simulink model "Seven_dof2024a_DK"  (R2025b)
settings: Solver=ode45  StartTime=0.0  StopTime=360  RelTol=1e-3
values from neighbouring files (symbols this model uses):
  Bf = 1.6    [Sensor_wz_u.m]    (also in unlinear_7DOF_Parameters.m)
  Br = 1.6    [Sensor_wz_u.m]    (also in unlinear_7DOF_Parameters.m)
  g = 9.8    [unlinear_7DOF_Parameters.m]
  hg = 0.5    [unlinear_7DOF_Parameters.m]
  i_sw = 20    [unlinear_7DOF_Parameters.m]
  L = Lf+Lr    (= 2.6)    [unlinear_7DOF_Parameters.m]
  Lf = 1.2    [Sensor_wz_u.m]    (also in unlinear_7DOF_Parameters.m)
  Lr = 1.4    [Sensor_wz_u.m]    (also in unlinear_7DOF_Parameters.m)
  mb = 1600    [unlinear_7DOF_Parameters.m]
  mw = (m-mb)/4    (= 41.25)    [unlinear_7DOF_Parameters.m]
  r = 0.354    [unlinear_7DOF_Parameters.m]
  u_fl = 0.3    [unlinear_7DOF_Parameters.m]
  u_fr = 0.8    [unlinear_7DOF_Parameters.m]
  u_rl = 0.3    [unlinear_7DOF_Parameters.m]
  u_rr = 0.8    [unlinear_7DOF_Parameters.m]
libraries: sharedTrackingLibrary x2, Solver_SF x1
settings Model: Creator=dzY  LastModifiedBy=odene
settings SolverCC: AlgebraicLoopSolver=TrustRegion
settings DataIOCC: LimitDataPoints=on  SaveFormat=Array  ReturnWorkspaceOutputs=off
settings OptimizationCC: BlockReduction=off  BooleanDataType=off  LifeSpan=inf
settings DebuggingCC: AlgebraicLoopMsg=none  SaveWithParameterizedLinksMsg=none  UnderspecifiedInitializationDetection=Classic  MergeDetectMultiDrivingBlocksExec=none  SignalResolutionControl=TryResolveAllWithWarning  UnconnectedInputMsg=warning  UnconnectedOutputMsg=warning  UnconnectedLineMsg=warning  SFUnexpectedBacktrackingDiag=warning  SFNoUnconditionalDefaultTransitionDiag=warning  SFExecutionAtInitializationDiag=none  ArithmeticOperatorsInVariantConditions=warning
settings HardwareCC: ProdBitPerPointer=32.0  ProdBitPerSizeT=32.0  ProdBitPerPtrDiffT=32.0  ProdLargestAtomicFloat=None  ProdIntDivRoundTo=Undefined  ProdEndianess=Unspecified  ProdWordSize=32.0  ProdHWDeviceType=32-bit Generic  TargetUnknown=on
settings ModelReferenceCC: EnableRefExpFcnMdlSchedulingChecks=on  PropagateSignalLabelsOutOfModel=off
settings SFSimCC: SimUseLocalCustomCode=off  CustomCodeUndefinedFunction=UseInterfaceOnly
settings RTWCC: RTWUseLocalCustomCode=off  GPUComputeCapability=3.5
settings CodeAppCC: StateflowObjectComments=on
settings GRTTargetCC: TargetLangStandard=C89/C90 (ANSI)
settings ConfigComp: CovMetricSettings=dw  CovSaveCumulativeToWorkspaceVar=on  CovSaveSingleToWorkspaceVar=on  CovExternalEMLEnable=off  CovSFcnEnable=off

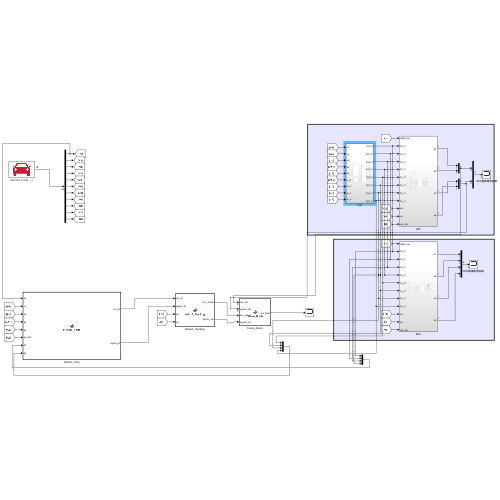
[thumbnail: Simulink's stored preview of the top-level diagram]
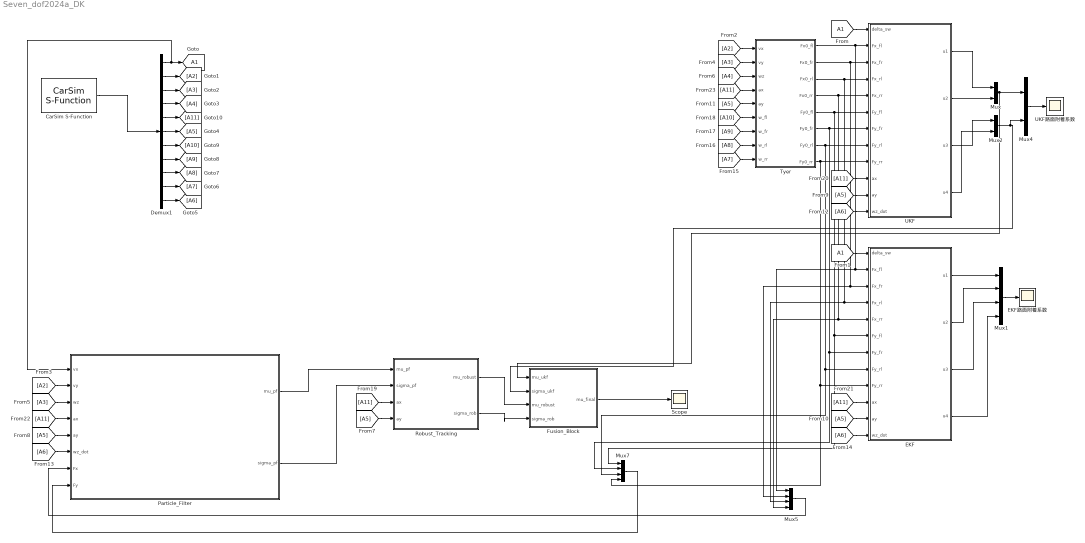
== system Seven_dof2024a_DK ==
  CarSim S-Function : Solver_SF/CarSim S-Function  Priority=1  VehicleCode=i_i  SIMFILE=simfile.sim
  Demux1 : Demux  Outputs=11
  EKF : Subsystem
  EKF路面附着系数 : Scope
      settings: ActiveDisplayYMinimum=0.13473  ActiveDisplayYMaximum=1.09614  DataLoggingSaveFormat=Array
  Fusion_Block : MATLAB Function  TreatAsAtomicUnit=on
  Mux : Mux  Inputs=2
  Mux1 : Mux
  Mux2 : Mux  Inputs=2
  Mux4 : Mux  Inputs=2
  Mux5 : Mux
  Mux7 : Mux
  Particle_Filter : MATLAB Function  TreatAsAtomicUnit=on
  Robust_Tracking : MATLAB Function  TreatAsAtomicUnit=on
  Scope : Scope
      settings: DataLoggingVariableName=ScopeData4
  Tyer : Subsystem
  UKF : Subsystem
  UKF路面附着系数 : Scope
      settings: ActiveDisplayYMinimum=0.13473  ActiveDisplayYMaximum=1.09614  DataLoggingSaveFormat=Array
  tag scope: A1=global
  wires:
  Mux4/1 -> UKF路面附着系数/1
  Tyer/1(Fx0_fl) -> Mux5/1, EKF/2(Fx_fl), UKF/2(Fx_fl)
  Tyer/2(Fx0_fr) -> Mux5/2, EKF/3(Fx_fr), UKF/3(Fx_fr)
  Tyer/3(Fx0_rl) -> Mux5/3, EKF/4(Fx_rl), UKF/4(Fx_rl)
  Tyer/4(Fx0_rr) -> Mux5/4, EKF/5(Fx_rr), UKF/5(Fx_rr)
  Tyer/5(Fy0_fl) -> Mux7/1, EKF/6(Fy_fl), UKF/6(Fy_fl)
  Tyer/6(Fy0_fr) -> Mux7/2, EKF/7(Fy_fr), UKF/7(Fy_fr)
  Tyer/7(Fy0_rl) -> Mux7/3, EKF/8(Fy_rl), UKF/8(Fy_rl)
  Tyer/8(Fy0_rr) -> Mux7/4, EKF/9(Fy_rr), UKF/9(Fy_rr)
  EKF/1(u1) -> Mux1/1
  EKF/2(u2) -> Mux1/2
  EKF/4(u4) -> Mux1/4
  EKF/3(u3) -> Mux1/3
  Mux1/1 -> EKF路面附着系数/1
  Fusion_Block/1(mu_final) -> Scope/1
  Mux5/1 -> Particle_Filter/7(Fx)
  Mux7/1 -> Particle_Filter/8(Fy)
  Particle_Filter/2(sigma_pf) -> Robust_Tracking/2(sigma_pf)
  Particle_Filter/1(mu_pf) -> Robust_Tracking/1(mu_pf)
  Robust_Tracking/2(sigma_rob) -> Fusion_Block/4(sigma_rob)
  Robust_Tracking/1(mu_robust) -> Fusion_Block/3(mu_robust)
  UKF/1(u1) -> Mux/1
  UKF/2(u2) -> Mux/2
  UKF/3(u3) -> Mux2/1
  UKF/4(u4) -> Mux2/2
  Mux/1 -> Fusion_Block/1(mu_ukf), Mux4/1
  Mux2/1 -> Fusion_Block/2(sigma_ukf), Mux4/2
  CarSim S-Function/1 -> Demux1/1
  Demux1/1 -> [A1], Particle_Filter/1(vx)
  [A1] -> UKF/1(delta_sw)
  [A1] -> EKF/1(delta_sw)
  Demux1/2 -> [A2]
  [A2] -> Tyer/1(vx)
  [A2] -> Particle_Filter/2(vy)
  Demux1/3 -> [A3]
  [A3] -> Tyer/2(vy)
  [A3] -> Particle_Filter/3(wz)
  Demux1/4 -> [A4]
  [A4] -> Tyer/3(wz)
  Demux1/6 -> [A5]
  [A5] -> Robust_Tracking/4(ay)
  [A5] -> Particle_Filter/5(ay)
  [A5] -> UKF/11(ay)
  [A5] -> EKF/11(ay)
  [A5] -> Tyer/5(ay)
  Demux1/11 -> [A6]
  [A6] -> UKF/12(wz_dot)
  [A6] -> Particle_Filter/6(wz_dot)
  [A6] -> EKF/12(wz_dot)
  Demux1/10 -> [A7]
  [A7] -> Tyer/9(w_rr)
  Demux1/9 -> [A8]
  [A8] -> Tyer/8(w_rl)
  Demux1/8 -> [A9]
  [A9] -> Tyer/7(w_fr)
  Demux1/7 -> [A10]
  [A10] -> Tyer/6(w_fl)
  Demux1/5 -> [A11]
  [A11] -> Robust_Tracking/3(ax)
  [A11] -> UKF/10(ax)
  [A11] -> EKF/10(ax)
  [A11] -> Particle_Filter/4(ax)
  [A11] -> Tyer/4(ax)

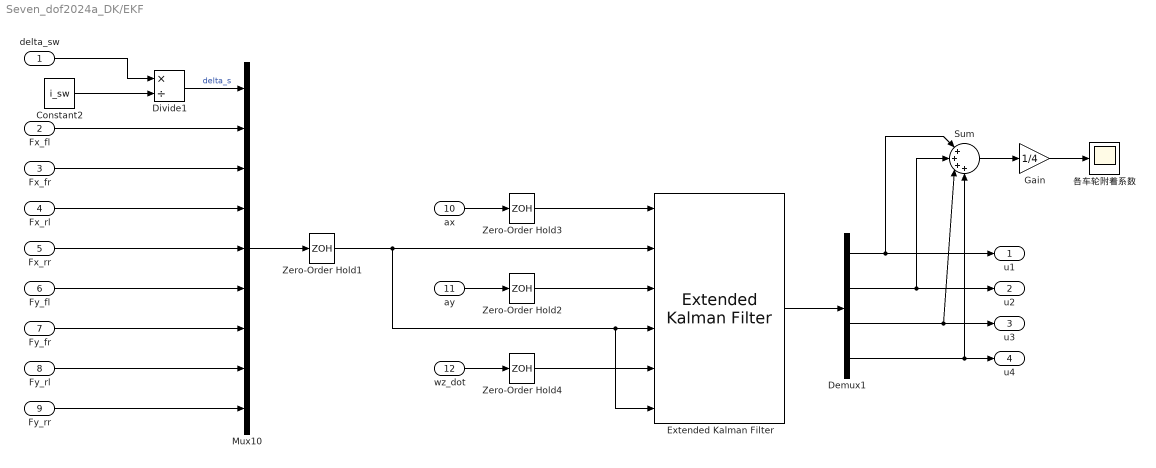
== system Seven_dof2024a_DK/EKF ==
  delta_sw : Inport
  Fx_fl : Inport  Port=2
  Fx_fr : Inport  Port=3
  Fx_rl : Inport  Port=4
  Fx_rr : Inport  Port=5
  Fy_fl : Inport  Port=6
  Fy_fr : Inport  Port=7
  Fy_rl : Inport  Port=8
  Fy_rr : Inport  Port=9
  ax : Inport  Port=10
  ay : Inport  Port=11
  wz_dot : Inport  Port=12
  Constant2 : Constant  Value=i_sw
  Demux1 : Demux
  Divide1 : Product  Inputs=*/
  Extended Kalman Filter : sharedTrackingLibrary/Extended Kalman Filter  StateTransitionFcn=LinearState_u  HasStateTransitionJacobianFcn=off  HasAdditiveProcessNoise=Additive  ProcessNoise=diag([0.1 0.1 0.1 0.1])  HasTimeVaryingProcessNoise=off  HasStateTransitionFcnExtraArgument=0  InitialState=[1;1; 1; 1]  InitialStateCovariance=1e-4  MeasurementFcn1=Sensor_ax_u  HasMeasurementJacobianFcn1=off  HasMeasurementEnablePort1=off  HasAdditiveMeasurementNoise1=Additive  MeasurementNoise1=0.0001  HasTimeVaryingMeasurementNoise1=off  HasMeasurementFcnExtraArgument1=1  HasMeasurementWrapping1=off  MeasurementFcn2=Sensor_ay_u  HasMeasurementJacobianFcn2=off  HasMeasurementEnablePort2=off  HasAdditiveMeasurementNoise2=Additive  MeasurementNoise2=0.0001  HasTimeVaryingMeasurementNoise2=off  HasMeasurementFcnExtraArgument2=1  HasMeasurementWrapping2=off  MeasurementFcn3=Sensor_wz_u  HasMeasurementJacobianFcn3=off  HasMeasurementEnablePort3=off  HasAdditiveMeasurementNoise3=Additive  MeasurementNoise3=0.0001  HasTimeVaryingMeasurementNoise3=off  HasMeasurementFcnExtraArgument3=1  HasMeasurementWrapping3=off  MeasurementFcn4=myMeasurementFcn  HasMeasurementJacobianFcn4=off  HasMeasurementEnablePort4=off  HasAdditiveMeasurementNoise4=Additive  MeasurementNoise4=1  HasTimeVaryingMeasurementNoise4=off  HasMeasurementFcnExtraArgument4=0  HasMeasurementWrapping4=off  MeasurementFcn5=myMeasurementFcn  HasMeasurementJacobianFcn5=off  HasMeasurementEnablePort5=off  HasAdditiveMeasurementNoise5=Additive  MeasurementNoise5=1  HasTimeVaryingMeasurementNoise5=off  HasMeasurementFcnExtraArgument5=0  HasMeasurementWrapping5=off  EnableMultirate=on  StateTransitionFcnSampleTime=0.01  MeasurementFcn1SampleTime=0.01  MeasurementFcn2SampleTime=0.01  MeasurementFcn3SampleTime=0.01  MeasurementFcn4SampleTime=1  MeasurementFcn5SampleTime=1  UseCurrentEstimator=on  OutputStateCovariance=off  DataType=double  SampleTime=0.01  NumberOfMeasurements=3
  Gain : Gain  Gain=1/4
  Mux10 : Mux  Inputs=9
  Sum : Sum  Inputs=|++++
  Zero-Order Hold{1..4} (4 alike) : ZeroOrderHold  SampleTime=0.01
  各车轮附着系数 : Scope
      settings: ActiveDisplayYMinimum=0.54572  ActiveDisplayYMaximum=0.55343
  u1 : Outport  VectorParamsAs1DForOutWhenUnconnected=off
  u2 : Outport  Port=2  VectorParamsAs1DForOutWhenUnconnected=off
  u3 : Outport  Port=3  VectorParamsAs1DForOutWhenUnconnected=off
  u4 : Outport  Port=4  VectorParamsAs1DForOutWhenUnconnected=off
  wires:
  Gain/1 -> 各车轮附着系数/1
  Sum/1 -> Gain/1
  Zero-Order Hold3/1 -> Extended Kalman Filter/1
  Zero-Order Hold2/1 -> Extended Kalman Filter/3
  Demux1/4 -> Sum/4, u4/1
  Zero-Order Hold1/1 -> Extended Kalman Filter/2, Extended Kalman Filter/6, Extended Kalman Filter/4
  Fy_rr/1 -> Mux10/9
  Fy_rl/1 -> Mux10/8
  Fy_fr/1 -> Mux10/7
  Fy_fl/1 -> Mux10/6
  Fx_rr/1 -> Mux10/5
  Fx_rl/1 -> Mux10/4
  Fx_fr/1 -> Mux10/3
  Fx_fl/1 -> Mux10/2
  Zero-Order Hold4/1 -> Extended Kalman Filter/5
  wz_dot/1 -> Zero-Order Hold4/1
  ay/1 -> Zero-Order Hold2/1
  ax/1 -> Zero-Order Hold3/1
  Constant2/1 -> Divide1/2
  delta_sw/1 -> Divide1/1
  Extended Kalman Filter/1 -> Demux1/1
  Mux10/1 -> Zero-Order Hold1/1
  Divide1/1 -> Mux10/1  "delta_s"
  Demux1/1 -> u1/1, Sum/1
  Demux1/3 -> Sum/3, u3/1
  Demux1/2 -> u2/1, Sum/2

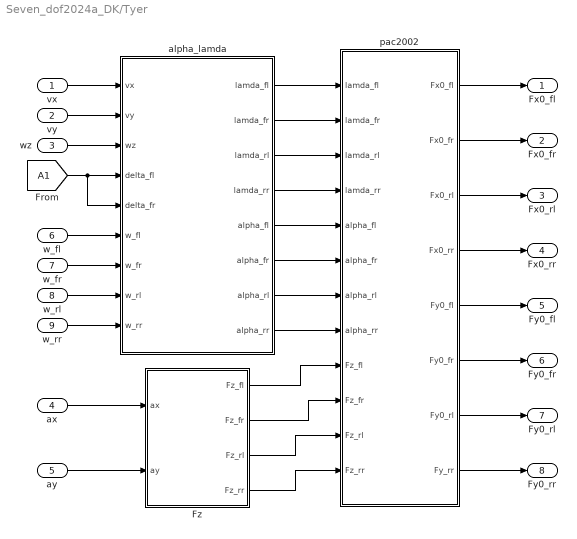
== system Seven_dof2024a_DK/Tyer ==
  vx : Inport
  vy : Inport  Port=2
  wz : Inport  Port=3
  ax : Inport  Port=4
  ay : Inport  Port=5
  w_fl : Inport  Port=6
  w_fr : Inport  Port=7
  w_rl : Inport  Port=8
  w_rr : Inport  Port=9
  Fz : Subsystem
  alpha_lamda : Subsystem
  pac2002 : Subsystem
  Fx0_fl : Outport  VectorParamsAs1DForOutWhenUnconnected=off
  Fx0_fr : Outport  Port=2  VectorParamsAs1DForOutWhenUnconnected=off
  Fx0_rl : Outport  Port=3  VectorParamsAs1DForOutWhenUnconnected=off
  Fx0_rr : Outport  Port=4  VectorParamsAs1DForOutWhenUnconnected=off
  Fy0_fl : Outport  Port=5  VectorParamsAs1DForOutWhenUnconnected=off
  Fy0_fr : Outport  Port=6  VectorParamsAs1DForOutWhenUnconnected=off
  Fy0_rl : Outport  Port=7  VectorParamsAs1DForOutWhenUnconnected=off
  Fy0_rr : Outport  Port=8  VectorParamsAs1DForOutWhenUnconnected=off
  wires:
  ay/1 -> Fz/2(ay)
  ax/1 -> Fz/1(ax)
  [A1] -> alpha_lamda/5(delta_fr), alpha_lamda/4(delta_fl)
  vx/1 -> alpha_lamda/1(vx)
  vy/1 -> alpha_lamda/2(vy)
  wz/1 -> alpha_lamda/3(wz)
  w_fl/1 -> alpha_lamda/6(w_fl)
  w_fr/1 -> alpha_lamda/7(w_fr)
  w_rl/1 -> alpha_lamda/8(w_rl)
  w_rr/1 -> alpha_lamda/9(w_rr)
  alpha_lamda/1(lamda_fl) -> pac2002/1(lamda_fl)
  alpha_lamda/2(lamda_fr) -> pac2002/2(lamda_fr)
  alpha_lamda/3(lamda_rl) -> pac2002/3(lamda_rl)
  alpha_lamda/4(lamda_rr) -> pac2002/4(lamda_rr)
  alpha_lamda/5(alpha_fl) -> pac2002/5(alpha_fl)
  alpha_lamda/6(alpha_fr) -> pac2002/6(alpha_fr)
  alpha_lamda/7(alpha_rl) -> pac2002/7(alpha_rl)
  alpha_lamda/8(alpha_rr) -> pac2002/8(alpha_rr)
  Fz/1(Fz_fl) -> pac2002/9(Fz_fl)
  Fz/2(Fz_fr) -> pac2002/10(Fz_fr)
  Fz/3(Fz_rl) -> pac2002/11(Fz_rl)
  Fz/4(Fz_rr) -> pac2002/12(Fz_rr)
  pac2002/1(Fx0_fl) -> Fx0_fl/1
  pac2002/2(Fx0_fr) -> Fx0_fr/1
  pac2002/3(Fx0_rl) -> Fx0_rl/1
  pac2002/4(Fx0_rr) -> Fx0_rr/1
  pac2002/5(Fy0_fl) -> Fy0_fl/1
  pac2002/6(Fy0_fr) -> Fy0_fr/1
  pac2002/7(Fy0_rl) -> Fy0_rl/1
  pac2002/8(Fy_rr) -> Fy0_rr/1

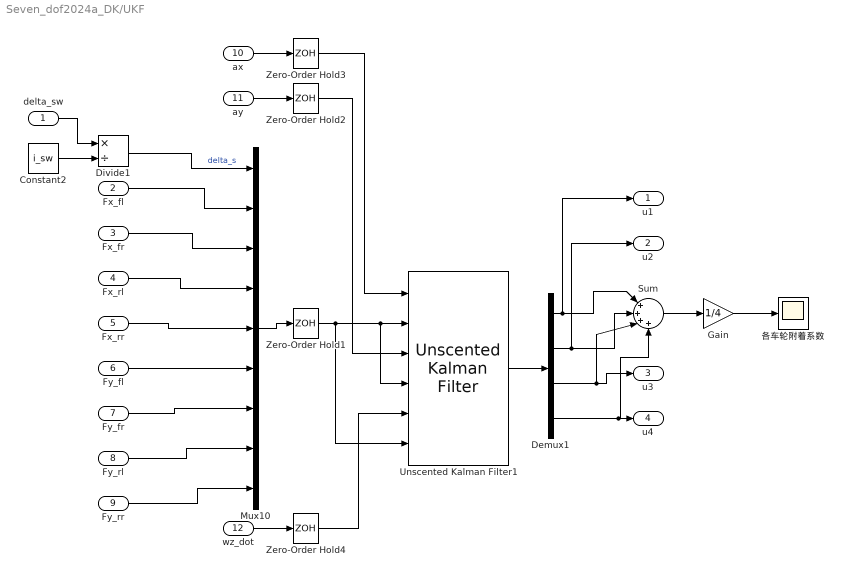
== system Seven_dof2024a_DK/UKF ==
  delta_sw : Inport
  Fx_fl : Inport  Port=2
  Fx_fr : Inport  Port=3
  Fx_rl : Inport  Port=4
  Fx_rr : Inport  Port=5
  Fy_fl : Inport  Port=6
  Fy_fr : Inport  Port=7
  Fy_rl : Inport  Port=8
  Fy_rr : Inport  Port=9
  ax : Inport  Port=10
  ay : Inport  Port=11
  wz_dot : Inport  Port=12
  Constant2 : Constant  Value=i_sw
  Demux1 : Demux
  Divide1 : Product  Inputs=*/
  Gain : Gain  Gain=1/4
  Mux10 : Mux  Inputs=9
  Sum : Sum  Inputs=|++++
  Unscented Kalman Filter1 : sharedTrackingLibrary/Unscented Kalman Filter  StateTransitionFcn=LinearState_u  HasAdditiveProcessNoise=Additive  ProcessNoise=diag([0.1 0.1 0.1 0.1])  HasTimeVaryingProcessNoise=off  HasStateTransitionFcnExtraArgument=0  InitialState=[1;1; 1; 1]  InitialStateCovariance=1e-4  Alpha=1e-3  Beta=2  Kappa=0  MeasurementFcn1=Sensor_ax_u  HasMeasurementEnablePort1=off  HasAdditiveMeasurementNoise1=Additive  MeasurementNoise1=0.0001  HasTimeVaryingMeasurementNoise1=off  HasMeasurementFcnExtraArgument1=1  HasMeasurementWrapping1=off  MeasurementFcn2=Sensor_ay_u  HasMeasurementEnablePort2=off  HasAdditiveMeasurementNoise2=Additive  MeasurementNoise2=0.0001  HasTimeVaryingMeasurementNoise2=off  HasMeasurementFcnExtraArgument2=1  HasMeasurementWrapping2=off  MeasurementFcn3=Sensor_wz_u  HasMeasurementEnablePort3=off  HasAdditiveMeasurementNoise3=Additive  MeasurementNoise3=0.0001  HasTimeVaryingMeasurementNoise3=off  HasMeasurementFcnExtraArgument3=1  HasMeasurementWrapping3=off  MeasurementFcn4=myMeasurementFcn  HasMeasurementEnablePort4=off  HasAdditiveMeasurementNoise4=Additive  MeasurementNoise4=1  HasTimeVaryingMeasurementNoise4=off  HasMeasurementFcnExtraArgument4=0  HasMeasurementWrapping4=off  MeasurementFcn5=myMeasurementFcn  HasMeasurementEnablePort5=off  HasAdditiveMeasurementNoise5=Additive  MeasurementNoise5=1  HasTimeVaryingMeasurementNoise5=off  HasMeasurementFcnExtraArgument5=0  HasMeasurementWrapping5=off  EnableMultirate=on  StateTransitionFcnSampleTime=0.01  MeasurementFcn1SampleTime=0.01  MeasurementFcn2SampleTime=0.01  MeasurementFcn3SampleTime=0.01  MeasurementFcn4SampleTime=1  MeasurementFcn5SampleTime=1  UseCurrentEstimator=on  OutputStateCovariance=off  DataType=double  SampleTime=1  NumberOfMeasurements=3
      link override Correct3/MATLAB System: SimulateUsing=Interpreted execution
  Zero-Order Hold{1..4} (4 alike) : ZeroOrderHold  SampleTime=0.01
  各车轮附着系数 : Scope
      settings: ActiveDisplayYMinimum=0.49277  ActiveDisplayYMaximum=1.05636
  u1 : Outport  VectorParamsAs1DForOutWhenUnconnected=off
  u2 : Outport  Port=2  VectorParamsAs1DForOutWhenUnconnected=off
  u3 : Outport  Port=3  VectorParamsAs1DForOutWhenUnconnected=off
  u4 : Outport  Port=4  VectorParamsAs1DForOutWhenUnconnected=off
  wires:
  Fx_fr/1 -> Mux10/3
  delta_sw/1 -> Divide1/1
  Fx_rr/1 -> Mux10/5
  Constant2/1 -> Divide1/2
  Zero-Order Hold4/1 -> Unscented Kalman Filter1/5
  Fy_fl/1 -> Mux10/6
  Fx_rl/1 -> Mux10/4
  Divide1/1 -> Mux10/1  "delta_s"
  Fx_fl/1 -> Mux10/2
  Fy_fr/1 -> Mux10/7
  Fy_rl/1 -> Mux10/8
  Fy_rr/1 -> Mux10/9
  ax/1 -> Zero-Order Hold3/1
  Sum/1 -> Gain/1
  ay/1 -> Zero-Order Hold2/1
  wz_dot/1 -> Zero-Order Hold4/1
  Zero-Order Hold3/1 -> Unscented Kalman Filter1/1
  Zero-Order Hold2/1 -> Unscented Kalman Filter1/3
  Zero-Order Hold1/1 -> Unscented Kalman Filter1/4, Unscented Kalman Filter1/2, Unscented Kalman Filter1/6
  Demux1/4 -> Sum/4, u4/1
  Unscented Kalman Filter1/1 -> Demux1/1
  Demux1/1 -> Sum/1, u1/1
  Demux1/2 -> Sum/2, u2/1
  Demux1/3 -> Sum/3, u3/1
  Gain/1 -> 各车轮附着系数/1
  Mux10/1 -> Zero-Order Hold1/1

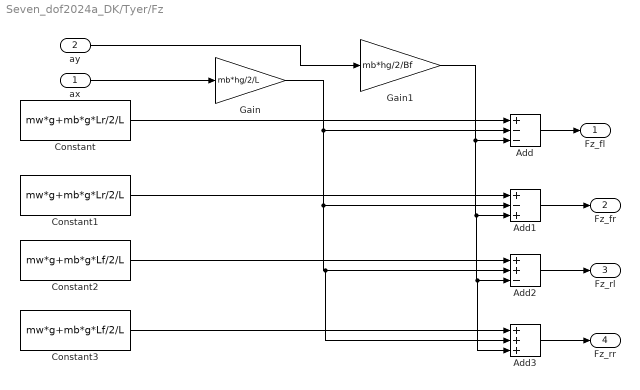
== system Seven_dof2024a_DK/Tyer/Fz ==
  ax : Inport
  ay : Inport  Port=2
  Add : Sum  Inputs=+--
  Add1 : Sum  Inputs=+-+
  Add2 : Sum  Inputs=++-
  Add3 : Sum  Inputs=+++
  Constant : Constant  Value=mw*g+mb*g*Lr/2/L
  Constant1 : Constant  Value=mw*g+mb*g*Lr/2/L
  Constant2 : Constant  Value=mw*g+mb*g*Lf/2/L
  Constant3 : Constant  Value=mw*g+mb*g*Lf/2/L
  Gain : Gain  Gain=mb*hg/2/L
  Gain1 : Gain  Gain=mb*hg/2/Bf
  Fz_fl : Outport  VectorParamsAs1DForOutWhenUnconnected=off
  Fz_fr : Outport  Port=2  VectorParamsAs1DForOutWhenUnconnected=off
  Fz_rl : Outport  Port=3  VectorParamsAs1DForOutWhenUnconnected=off
  Fz_rr : Outport  Port=4  VectorParamsAs1DForOutWhenUnconnected=off
  wires:
  Constant1/1 -> Add1/1
  Constant2/1 -> Add2/1
  Constant/1 -> Add/1
  Gain/1 -> Add3/2, Add2/2, Add1/2, Add/2
  Gain1/1 -> Add3/3, Add2/3, Add1/3, Add/3
  Constant3/1 -> Add3/1
  ay/1 -> Gain1/1
  ax/1 -> Gain/1
  Add3/1 -> Fz_rr/1
  Add2/1 -> Fz_rl/1
  Add1/1 -> Fz_fr/1
  Add/1 -> Fz_fl/1

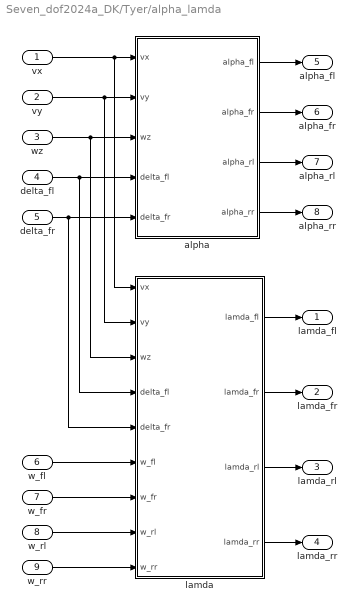
== system Seven_dof2024a_DK/Tyer/alpha_lamda ==
  vx : Inport
  vy : Inport  Port=2
  wz : Inport  Port=3
  delta_fl : Inport  Port=4
  delta_fr : Inport  Port=5
  w_fl : Inport  Port=6
  w_fr : Inport  Port=7
  w_rl : Inport  Port=8
  w_rr : Inport  Port=9
  alpha : Subsystem
  lamda : Subsystem
  lamda_fl : Outport  VectorParamsAs1DForOutWhenUnconnected=off
  lamda_fr : Outport  Port=2  VectorParamsAs1DForOutWhenUnconnected=off
  lamda_rl : Outport  Port=3  VectorParamsAs1DForOutWhenUnconnected=off
  lamda_rr : Outport  Port=4  VectorParamsAs1DForOutWhenUnconnected=off
  alpha_fl : Outport  Port=5  VectorParamsAs1DForOutWhenUnconnected=off
  alpha_fr : Outport  Port=6  VectorParamsAs1DForOutWhenUnconnected=off
  alpha_rl : Outport  Port=7  VectorParamsAs1DForOutWhenUnconnected=off
  alpha_rr : Outport  Port=8  VectorParamsAs1DForOutWhenUnconnected=off
  wires:
  lamda/3(lamda_rl) -> lamda_rl/1
  lamda/4(lamda_rr) -> lamda_rr/1
  lamda/2(lamda_fr) -> lamda_fr/1
  lamda/1(lamda_fl) -> lamda_fl/1
  w_rr/1 -> lamda/9(w_rr)
  w_rl/1 -> lamda/8(w_rl)
  w_fr/1 -> lamda/7(w_fr)
  w_fl/1 -> lamda/6(w_fl)
  delta_fr/1 -> alpha/5(delta_fr), lamda/5(delta_fr)
  delta_fl/1 -> alpha/4(delta_fl), lamda/4(delta_fl)
  wz/1 -> alpha/3(wz), lamda/3(wz)
  vy/1 -> alpha/2(vy), lamda/2(vy)
  vx/1 -> alpha/1(vx), lamda/1(vx)
  alpha/4(alpha_rr) -> alpha_rr/1
  alpha/3(alpha_rl) -> alpha_rl/1
  alpha/2(alpha_fr) -> alpha_fr/1
  alpha/1(alpha_fl) -> alpha_fl/1

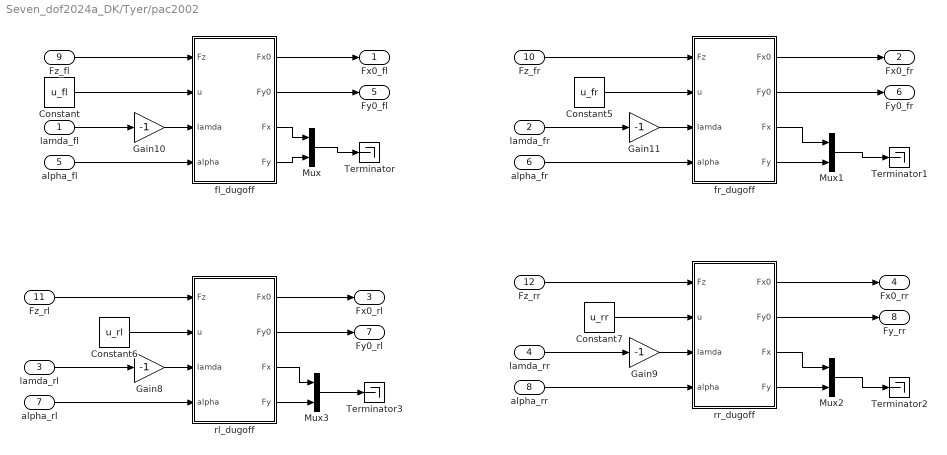
== system Seven_dof2024a_DK/Tyer/pac2002 ==
  lamda_fl : Inport
  lamda_fr : Inport  Port=2
  lamda_rl : Inport  Port=3
  lamda_rr : Inport  Port=4
  alpha_fl : Inport  Port=5
  alpha_fr : Inport  Port=6
  alpha_rl : Inport  Port=7
  alpha_rr : Inport  Port=8
  Fz_fl : Inport  Port=9
  Fz_fr : Inport  Port=10
  Fz_rl : Inport  Port=11
  Fz_rr : Inport  Port=12
  Constant : Constant  Value=u_fl
  Constant5 : Constant  Value=u_fr
  Constant6 : Constant  Value=u_rl
  Constant7 : Constant  Value=u_rr
  Gain{8..11} (4 alike) : Gain  Gain=-1
  Mux{,1..3} (4 alike) : Mux  Inputs=2
  Terminator{,1..3} (4 alike) : Terminator
  fl_dugoff : MATLAB Function  TreatAsAtomicUnit=on
  fr_dugoff : MATLAB Function  TreatAsAtomicUnit=on
  rl_dugoff : MATLAB Function  TreatAsAtomicUnit=on
  rr_dugoff : MATLAB Function  TreatAsAtomicUnit=on
  Fx0_fl : Outport  VectorParamsAs1DForOutWhenUnconnected=off
  Fx0_fr : Outport  Port=2  VectorParamsAs1DForOutWhenUnconnected=off
  Fx0_rl : Outport  Port=3  VectorParamsAs1DForOutWhenUnconnected=off
  Fx0_rr : Outport  Port=4  VectorParamsAs1DForOutWhenUnconnected=off
  Fy0_fl : Outport  Port=5  VectorParamsAs1DForOutWhenUnconnected=off
  Fy0_fr : Outport  Port=6  VectorParamsAs1DForOutWhenUnconnected=off
  Fy0_rl : Outport  Port=7  VectorParamsAs1DForOutWhenUnconnected=off
  Fy_rr : Outport  Port=8  VectorParamsAs1DForOutWhenUnconnected=off
  wires:
  alpha_fl/1 -> fl_dugoff/4(alpha)
  Fz_fl/1 -> fl_dugoff/1(Fz)
  Fz_rl/1 -> rl_dugoff/1(Fz)
  alpha_rr/1 -> rr_dugoff/4(alpha)
  Fz_rr/1 -> rr_dugoff/1(Fz)
  Constant/1 -> fl_dugoff/2(u)
  Fz_fr/1 -> fr_dugoff/1(Fz)
  Constant5/1 -> fr_dugoff/2(u)
  alpha_fr/1 -> fr_dugoff/4(alpha)
  Constant6/1 -> rl_dugoff/2(u)
  Constant7/1 -> rr_dugoff/2(u)
  lamda_fr/1 -> Gain11/1
  lamda_rl/1 -> Gain8/1
  lamda_rr/1 -> Gain9/1
  lamda_fl/1 -> Gain10/1
  fl_dugoff/1(Fx0) -> Fx0_fl/1
  rl_dugoff/1(Fx0) -> Fx0_rl/1
  fl_dugoff/2(Fy0) -> Fy0_fl/1
  fr_dugoff/2(Fy0) -> Fy0_fr/1
  rl_dugoff/2(Fy0) -> Fy0_rl/1
  rr_dugoff/2(Fy0) -> Fy_rr/1
  rr_dugoff/1(Fx0) -> Fx0_rr/1
  alpha_rl/1 -> rl_dugoff/4(alpha)
  Gain8/1 -> rl_dugoff/3(lamda)
  Gain9/1 -> rr_dugoff/3(lamda)
  Gain10/1 -> fl_dugoff/3(lamda)
  Gain11/1 -> fr_dugoff/3(lamda)
  fr_dugoff/1(Fx0) -> Fx0_fr/1
  fl_dugoff/3(Fx) -> Mux/1
  fl_dugoff/4(Fy) -> Mux/2
  Mux/1 -> Terminator/1
  Mux1/1 -> Terminator1/1
  fr_dugoff/3(Fx) -> Mux1/1
  fr_dugoff/4(Fy) -> Mux1/2
  rr_dugoff/3(Fx) -> Mux2/1
  rr_dugoff/4(Fy) -> Mux2/2
  Mux2/1 -> Terminator2/1
  rl_dugoff/3(Fx) -> Mux3/1
  rl_dugoff/4(Fy) -> Mux3/2
  Mux3/1 -> Terminator3/1

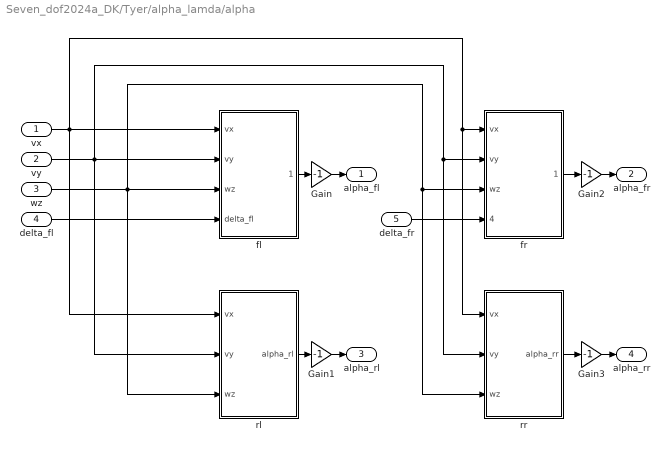
== system Seven_dof2024a_DK/Tyer/alpha_lamda/alpha ==
  vx : Inport
  vy : Inport  Port=2
  wz : Inport  Port=3
  delta_fl : Inport  Port=4
  delta_fr : Inport  Port=5
  Gain{,1..3} (4 alike) : Gain  Gain=-1
  fl : Subsystem
  fr : Subsystem
  rl : Subsystem
  rr : Subsystem
  alpha_fl : Outport  VectorParamsAs1DForOutWhenUnconnected=off
  alpha_fr : Outport  Port=2  VectorParamsAs1DForOutWhenUnconnected=off
  alpha_rl : Outport  Port=3  VectorParamsAs1DForOutWhenUnconnected=off
  alpha_rr : Outport  Port=4  VectorParamsAs1DForOutWhenUnconnected=off
  wires:
  delta_fr/1 -> fr/4(delta_fr)
  delta_fl/1 -> fl/4(delta_fl)
  vy/1 -> rl/2(vy), fl/2(vy), fr/2(vy), rr/2(vy)
  vx/1 -> rl/1(vx), fl/1(vx), fr/1(vx), rr/1(vx)
  wz/1 -> rl/3(wz), fr/3(wz), rr/3(wz), fl/3(wz)
  fl/1(alpha_fl) -> Gain/1
  Gain/1 -> alpha_fl/1
  rl/1(alpha_rl) -> Gain1/1
  Gain1/1 -> alpha_rl/1
  fr/1(alpha_fr) -> Gain2/1
  Gain2/1 -> alpha_fr/1
  rr/1(alpha_rr) -> Gain3/1
  Gain3/1 -> alpha_rr/1

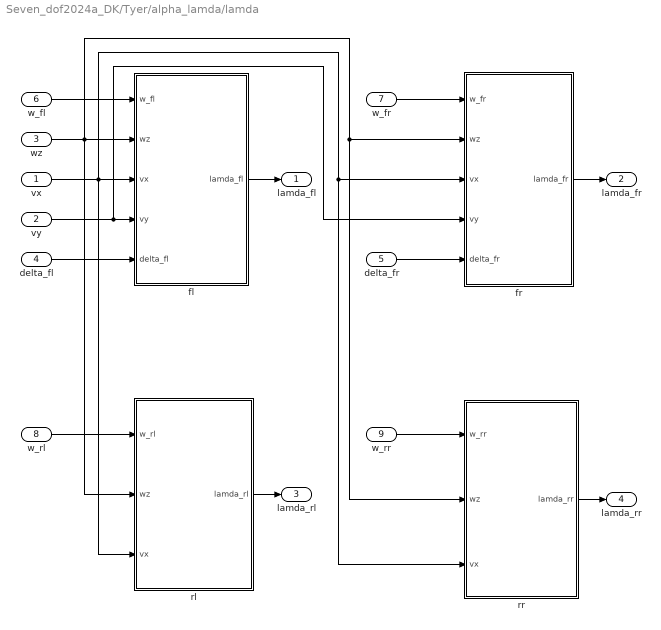
== system Seven_dof2024a_DK/Tyer/alpha_lamda/lamda ==
  vx : Inport
  vy : Inport  Port=2
  wz : Inport  Port=3
  delta_fl : Inport  Port=4
  delta_fr : Inport  Port=5
  w_fl : Inport  Port=6
  w_fr : Inport  Port=7
  w_rl : Inport  Port=8
  w_rr : Inport  Port=9
  fl : Subsystem
  fr : Subsystem
  rl : Subsystem
  rr : Subsystem
  lamda_fl : Outport  VectorParamsAs1DForOutWhenUnconnected=off
  lamda_fr : Outport  Port=2  VectorParamsAs1DForOutWhenUnconnected=off
  lamda_rl : Outport  Port=3  VectorParamsAs1DForOutWhenUnconnected=off
  lamda_rr : Outport  Port=4  VectorParamsAs1DForOutWhenUnconnected=off
  wires:
  fr/1(lamda_fr) -> lamda_fr/1
  rr/1(lamda_rr) -> lamda_rr/1
  w_rl/1 -> rl/1(w_rl)
  w_rr/1 -> rr/1(w_rr)
  w_fr/1 -> fr/1(w_fr)
  delta_fr/1 -> fr/5(delta_fr)
  delta_fl/1 -> fl/5(delta_fl)
  vy/1 -> fl/4(vy), fr/4(vy)
  vx/1 -> fl/3(vx), fr/3(vx), rr/3(vx), rl/3(vx)
  wz/1 -> fl/2(wz), fr/2(wz), rr/2(wz), rl/2(wz)
  w_fl/1 -> fl/1(w_fl)
  rl/1(lamda_rl) -> lamda_rl/1
  fl/1(lamda_fl) -> lamda_fl/1

== system Seven_dof2024a_DK/Tyer/alpha_lamda/alpha/fl ==
  vx : Inport
  vy : Inport  Port=2
  wz : Inport  Port=3
  delta_fl : Inport  Port=4
  Add2 : Sum
  Add3 : Sum  Inputs=+-
  Add4 : Sum  Inputs=-+
  Divide : Product  Inputs=/*
  Gain3 : Gain  Gain=Lf
  Gain4 : Gain  Gain=0.5*Bf
  Trigonometric Function : Trigonometry  Operator=atan
  alpha_fl : Outport  VectorParamsAs1DForOutWhenUnconnected=off
  wires:
  wz/1 -> Gain3/1, Gain4/1
  Add4/1 -> alpha_fl/1
  vy/1 -> Add2/1
  delta_fl/1 -> Add4/2
  vx/1 -> Add3/1
  Trigonometric Function/1 -> Add4/1
  Divide/1 -> Trigonometric Function/1
  Add3/1 -> Divide/1
  Add2/1 -> Divide/2
  Gain4/1 -> Add3/2
  Gain3/1 -> Add2/2

== system Seven_dof2024a_DK/Tyer/alpha_lamda/alpha/fr ==
  vx : Inport
  vy : Inport  Port=2
  wz : Inport  Port=3
  delta_fr : Inport  Port=4
  Add2 : Sum
  Add3 : Sum
  Add4 : Sum  Inputs=-+
  Divide : Product  Inputs=/*
  Gain3 : Gain  Gain=Lf
  Gain4 : Gain  Gain=0.5*Bf
  Trigonometric Function : Trigonometry  Operator=atan
  alpha_fr : Outport  VectorParamsAs1DForOutWhenUnconnected=off
  wires:
  Gain3/1 -> Add2/2
  Add2/1 -> Divide/2
  Add3/1 -> Divide/1
  Divide/1 -> Trigonometric Function/1
  Trigonometric Function/1 -> Add4/1
  vx/1 -> Add3/1
  delta_fr/1 -> Add4/2
  vy/1 -> Add2/1
  Add4/1 -> alpha_fr/1
  wz/1 -> Gain4/1, Gain3/1
  Gain4/1 -> Add3/2

== system Seven_dof2024a_DK/Tyer/alpha_lamda/alpha/rl ==
  vx : Inport
  vy : Inport  Port=2
  wz : Inport  Port=3
  Add2 : Sum  Inputs=+-
  Add3 : Sum  Inputs=+-
  Divide : Product  Inputs=/*
  Gain1 : Gain  Gain=-1
  Gain3 : Gain  Gain=Lr
  Gain4 : Gain  Gain=0.5*Br
  Trigonometric Function : Trigonometry  Operator=atan
  alpha_rl : Outport  VectorParamsAs1DForOutWhenUnconnected=off
  wires:
  Gain3/1 -> Add2/2
  Add2/1 -> Divide/2
  Add3/1 -> Divide/1
  Divide/1 -> Trigonometric Function/1
  vx/1 -> Add3/1
  vy/1 -> Add2/1
  wz/1 -> Gain4/1, Gain3/1
  Trigonometric Function/1 -> Gain1/1
  Gain4/1 -> Add3/2
  Gain1/1 -> alpha_rl/1

== system Seven_dof2024a_DK/Tyer/alpha_lamda/alpha/rr ==
  vx : Inport
  vy : Inport  Port=2
  wz : Inport  Port=3
  Add2 : Sum  Inputs=+-
  Add3 : Sum
  Divide : Product  Inputs=/*
  Gain2 : Gain  Gain=-1
  Gain3 : Gain  Gain=Lr
  Gain4 : Gain  Gain=0.5*Br
  Trigonometric Function : Trigonometry  Operator=atan
  alpha_rr : Outport  VectorParamsAs1DForOutWhenUnconnected=off
  wires:
  Trigonometric Function/1 -> Gain2/1
  wz/1 -> Gain3/1, Gain4/1
  vy/1 -> Add2/1
  vx/1 -> Add3/1
  Divide/1 -> Trigonometric Function/1
  Add3/1 -> Divide/1
  Add2/1 -> Divide/2
  Gain3/1 -> Add2/2
  Gain4/1 -> Add3/2
  Gain2/1 -> alpha_rr/1

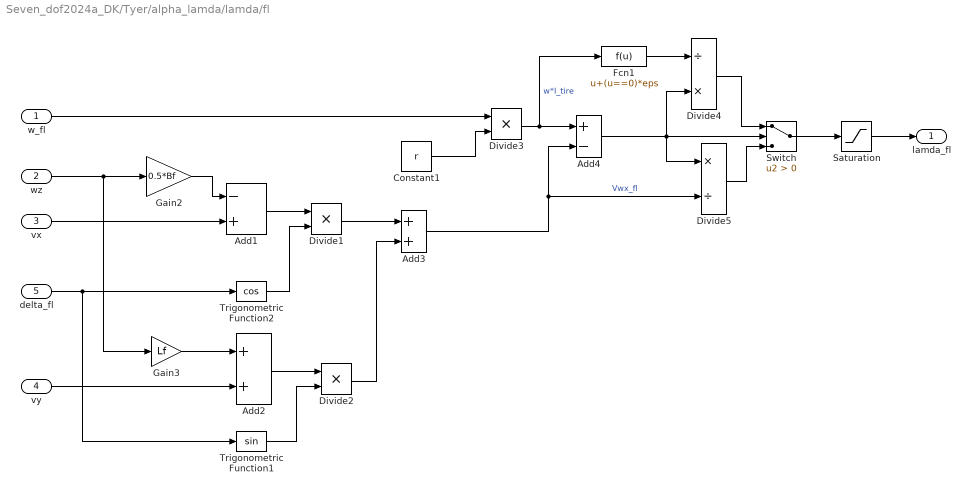
== system Seven_dof2024a_DK/Tyer/alpha_lamda/lamda/fl ==
  w_fl : Inport
  wz : Inport  Port=2
  vx : Inport  Port=3
  vy : Inport  Port=4
  delta_fl : Inport  Port=5
  Add1 : Sum  Inputs=-+
  Add2 : Sum
  Add3 : Sum
  Add4 : Sum  Inputs=+-
  Constant1 : Constant  Value=r
  Divide1 : Product  Inputs=**
  Divide2 : Product  Inputs=**
  Divide3 : Product  Inputs=**
  Divide4 : Product  Inputs=/*
  Divide5 : Product  Inputs=*/
  Fcn1 : Fcn  Expr=u+(u==0)*eps
  Gain2 : Gain  Gain=0.5*Bf
  Gain3 : Gain  Gain=Lf
  Saturation : Saturate  UpperLimit=1  LowerLimit=-1
  Switch : Switch  Criteria=u2 > Threshold  SaturateOnIntegerOverflow=off  InputSameDT=off
  Trigonometric Function1 : Trigonometry
  Trigonometric Function2 : Trigonometry  Operator=cos
  lamda_fl : Outport  VectorParamsAs1DForOutWhenUnconnected=off
  wires:
  Switch/1 -> Saturation/1
  Add3/1 -> Add4/2, Divide5/2  "Vwx_fl"
  Add4/1 -> Switch/2, Divide4/2, Divide5/1
  Divide4/1 -> Switch/1
  Divide5/1 -> Switch/3
  Fcn1/1 -> Divide4/1
  vx/1 -> Add1/2
  Gain2/1 -> Add1/1
  wz/1 -> Gain3/1, Gain2/1
  Add1/1 -> Divide1/1
  delta_fl/1 -> Trigonometric Function2/1, Trigonometric Function1/1
  Trigonometric Function2/1 -> Divide1/2
  vy/1 -> Add2/2
  Gain3/1 -> Add2/1
  Add2/1 -> Divide2/1
  Trigonometric Function1/1 -> Divide2/2
  Divide1/1 -> Add3/1
  Divide2/1 -> Add3/2
  w_fl/1 -> Divide3/1
  Constant1/1 -> Divide3/2
  Divide3/1 -> Add4/1, Fcn1/1  "w*I_tire"
  Saturation/1 -> lamda_fl/1

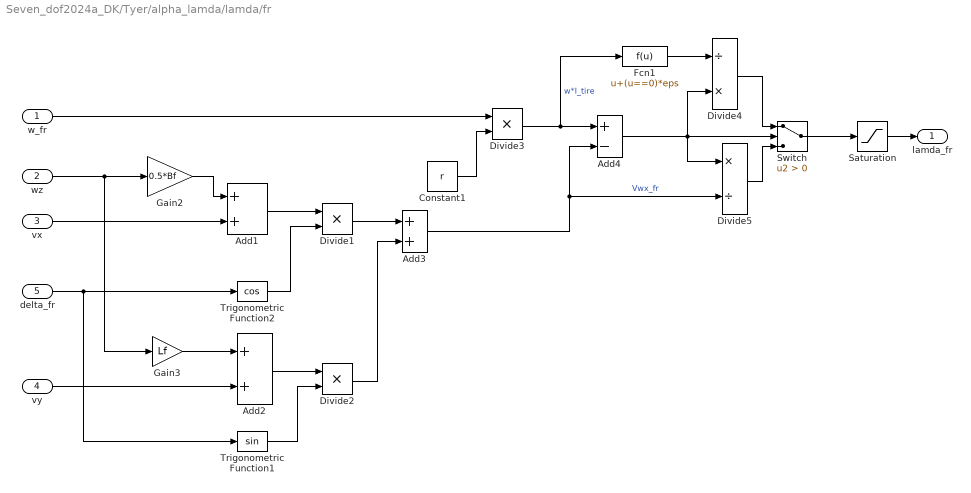
== system Seven_dof2024a_DK/Tyer/alpha_lamda/lamda/fr ==
  w_fr : Inport
  wz : Inport  Port=2
  vx : Inport  Port=3
  vy : Inport  Port=4
  delta_fr : Inport  Port=5
  Add1 : Sum
  Add2 : Sum
  Add3 : Sum
  Add4 : Sum  Inputs=+-
  Constant1 : Constant  Value=r
  Divide1 : Product  Inputs=**
  Divide2 : Product  Inputs=**
  Divide3 : Product  Inputs=**
  Divide4 : Product  Inputs=/*
  Divide5 : Product  Inputs=*/
  Fcn1 : Fcn  Expr=u+(u==0)*eps
  Gain2 : Gain  Gain=0.5*Bf
  Gain3 : Gain  Gain=Lf
  Saturation : Saturate  UpperLimit=1  LowerLimit=-1
  Switch : Switch  Criteria=u2 > Threshold  SaturateOnIntegerOverflow=off  InputSameDT=off
  Trigonometric Function1 : Trigonometry
  Trigonometric Function2 : Trigonometry  Operator=cos
  lamda_fr : Outport  VectorParamsAs1DForOutWhenUnconnected=off
  wires:
  Saturation/1 -> lamda_fr/1
  vx/1 -> Add1/2
  Gain2/1 -> Add1/1
  wz/1 -> Gain3/1, Gain2/1
  Add1/1 -> Divide1/1
  delta_fr/1 -> Trigonometric Function2/1, Trigonometric Function1/1
  Trigonometric Function2/1 -> Divide1/2
  vy/1 -> Add2/2
  Gain3/1 -> Add2/1
  Add2/1 -> Divide2/1
  Trigonometric Function1/1 -> Divide2/2
  Divide1/1 -> Add3/1
  Divide2/1 -> Add3/2
  w_fr/1 -> Divide3/1
  Constant1/1 -> Divide3/2
  Divide3/1 -> Fcn1/1, Add4/1  "w*I_tire"
  Fcn1/1 -> Divide4/1
  Divide5/1 -> Switch/3
  Divide4/1 -> Switch/1
  Add4/1 -> Divide5/1, Divide4/2, Switch/2
  Add3/1 -> Divide5/2, Add4/2  "Vwx_fr"
  Switch/1 -> Saturation/1

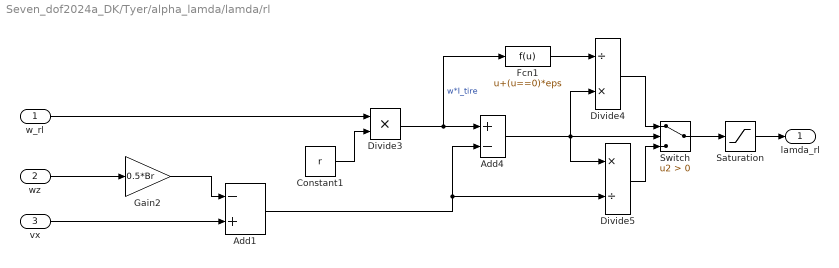
== system Seven_dof2024a_DK/Tyer/alpha_lamda/lamda/rl ==
  w_rl : Inport
  wz : Inport  Port=2
  vx : Inport  Port=3
  Add1 : Sum  Inputs=-+
  Add4 : Sum  Inputs=+-
  Constant1 : Constant  Value=r
  Divide3 : Product  Inputs=**
  Divide4 : Product  Inputs=/*
  Divide5 : Product  Inputs=*/
  Fcn1 : Fcn  Expr=u+(u==0)*eps
  Gain2 : Gain  Gain=0.5*Br
  Saturation : Saturate  UpperLimit=1  LowerLimit=-1
  Switch : Switch  Criteria=u2 > Threshold  SaturateOnIntegerOverflow=off  InputSameDT=off
  lamda_rl : Outport  VectorParamsAs1DForOutWhenUnconnected=off
  wires:
  Saturation/1 -> lamda_rl/1
  vx/1 -> Add1/2
  Gain2/1 -> Add1/1
  wz/1 -> Gain2/1
  w_rl/1 -> Divide3/1
  Constant1/1 -> Divide3/2
  Divide3/1 -> Fcn1/1, Add4/1  "w*I_tire"
  Fcn1/1 -> Divide4/1
  Divide5/1 -> Switch/3
  Divide4/1 -> Switch/1
  Add4/1 -> Divide5/1, Divide4/2, Switch/2
  Add1/1 -> Divide5/2, Add4/2
  Switch/1 -> Saturation/1

== system Seven_dof2024a_DK/Tyer/alpha_lamda/lamda/rr ==
  w_rr : Inport
  wz : Inport  Port=2
  vx : Inport  Port=3
  Add1 : Sum
  Add4 : Sum  Inputs=+-
  Constant1 : Constant  Value=r
  Divide3 : Product  Inputs=**
  Divide4 : Product  Inputs=/*
  Divide5 : Product  Inputs=*/
  Fcn1 : Fcn  Expr=u+(u==0)*eps
  Gain2 : Gain  Gain=0.5*Br
  Saturation : Saturate  UpperLimit=1  LowerLimit=-1
  Switch : Switch  Criteria=u2 > Threshold  SaturateOnIntegerOverflow=off  InputSameDT=off
  lamda_rr : Outport  VectorParamsAs1DForOutWhenUnconnected=off
  wires:
  Saturation/1 -> lamda_rr/1
  Switch/1 -> Saturation/1
  Constant1/1 -> Divide3/2
  w_rr/1 -> Divide3/1
  wz/1 -> Gain2/1
  Gain2/1 -> Add1/1
  vx/1 -> Add1/2
  Divide3/1 -> Fcn1/1, Add4/1  "w*I_tire"
  Fcn1/1 -> Divide4/1
  Divide5/1 -> Switch/3
  Divide4/1 -> Switch/1
  Add4/1 -> Divide5/1, Divide4/2, Switch/2
  Add1/1 -> Divide5/2, Add4/2  "Vwx_rr"

== matlab function Seven_dof2024a_DK/Robust_Tracking ==
  data: mu_pf input; mu_robust output; sigma_pf input; ax input; ay input; sigma_rob output
function [mu_robust, sigma_rob] = Robust_Tracking(mu_pf, sigma_pf, ax, ay)
%#codegen

persistent mu_est P

% Initialize
if isempty(mu_est)
    mu_est = 0.7;
    P      = 0.1;
end

% --- Process noise (adaptive) ---
Q = 0.001;
innovation = mu_pf - mu_est;
if abs(innovation) > 0.1
    Q = Q * 5; % increase noise if sudden change detected
end

% --- Predict ---
mu_pred = mu_est;
P_pred  = P + Q;

% --- Huber likelihood (robust to outliers) ---
delta = 0.05;
if abs(innovation) <= delta
    K = P_pred / (P_pred + sigma_pf^2 + 1e-6);
else
    K = P_pred / (P_pred + sigma_pf^2 + 1e-6) * delta / abs(innovation);
end

% --- Update ---
mu_est = mu_pred + K * innovation;
P      = (1 - K) * P_pred;

% Clamp
mu_est = max(0.1, min(1.0, mu_est));

% --- Output ---
mu_robust = mu_est;
sigma_rob = sqrt(P);

== matlab function Seven_dof2024a_DK/Particle_Filter ==
  data: vx input; mu_pf output; vy input; wz input; ax input; ay input; wz_dot input; Fx input; Fy input; sigma_pf output
function [mu_pf, sigma_pf] = Particle_Filter(vx, vy, wz, ax, ay, wz_dot, Fx, Fy)
%#codegen

persistent particles weights N

% Initialize on first run
if isempty(particles)
    N = int32(500);
    particles = 0.4 + 0.6 * rand(1, 500);
    weights   = ones(1, 500) / 500;
end

% --- Prediction: add process noise ---
particles = particles + 0.01 * randn(1, 500);
particles = max(0.1, min(1.0, particles));

% --- Measurement: use lateral acceleration ---
m = 1500;
Fy_meas = m * ay;
Fy_pred_all = particles * m * 9.81;

% --- Update weights ---
R = 500;
likelihood = exp(-0.5 * ((Fy_meas - Fy_pred_all).^2) / R);
weights = weights .* likelihood;
weights = weights / (sum(weights) + 1e-10);

% --- Resample ---
cumW = cumsum(weights);
positions = ((0:499) + rand) / 500;
newParticles = zeros(1, 500);
i = 1;
for j = 1:500
    while positions(j) > cumW(i) && i < 500
        i = i + 1;
    end
    newParticles(j) = particles(i);
end
particles = newParticles;
weights   = ones(1, 500) / 500;

% --- Output ---
mu_pf    = sum(weights .* particles);
sigma_pf = sqrt(sum(weights .* (particles - mu_pf).^2));

== matlab function Seven_dof2024a_DK/Fusion_Block ==
  data: mu_ukf input; mu_final output; sigma_ukf input; mu_robust input; sigma_rob input
function mu_final = Fusion_Block(mu_ukf, sigma_ukf, mu_robust, sigma_rob)
%#codegen
mu_final = double(0);
s1 = double(sigma_ukf);
s2 = double(sigma_rob);
w1 = 1 / (s1(1) * s1(1) + 1e-6);
w2 = 1 / (s2(1) * s2(1) + 1e-6);
m1 = double(mu_ukf);
m2 = double(mu_robust);
mu_final = (w1 * m1(1) + w2 * m2(1)) / (w1 + w2);
if mu_final < 0.1
mu_final = 0.1;
elseif mu_final > 1.0
mu_final = 1.0;
end

== matlab function Seven_dof2024a_DK/Tyer/pac2002/fl_dugoff ==
  data: Fz input; Fx0 output; u input; lamda input; alpha input; Fy0 output; Fx output; Fy output
function [Fx0,Fy0,Fx,Fy] = tire(Fz,u,lamda,alpha)
cx = -20;
cy = -20;
L = (1-lamda)/(2*sqrt((cx^2)*(lamda^2)+(cy^2)*((tan(alpha))^2)));
if L<1
    fL = L*(2-L);
else
    fL = 1;
end
Fx0 = Fz*cx*lamda*fL/(1-lamda);
Fy0 = Fz*cy*tan(alpha)*fL/(1-lamda);
Fx = u*Fx0;
Fy = u*Fy0;

== matlab function Seven_dof2024a_DK/Tyer/pac2002/fr_dugoff ==
  data: Fz input; Fx0 output; u input; lamda input; alpha input; Fy0 output; Fx output; Fy output
function [Fx0,Fy0,Fx,Fy] = tire(Fz,u,lamda,alpha)
cx = -20;
cy = -20;
L = (1-lamda)/(2*sqrt((cx^2)*(lamda^2)+(cy^2)*((tan(alpha))^2)));
if L<1
    fL = L*(2-L);
else
    fL = 1;
end
Fx0 = Fz*cx*lamda*fL/(1-lamda);
Fy0 = Fz*cy*tan(alpha)*fL/(1-lamda);
Fx = u*Fx0;
Fy = u*Fy0;

== matlab function Seven_dof2024a_DK/Tyer/pac2002/rl_dugoff ==
  data: Fz input; Fx0 output; u input; lamda input; alpha input; Fy0 output; Fx output; Fy output
function [Fx0,Fy0,Fx,Fy] = tire(Fz,u,lamda,alpha)
cx = -20;
cy = -20;
L = (1-lamda)/(2*sqrt(cx^2*lamda^2+cy^2*(tan(alpha))^2));
if L<1
    fL = L*(2-L);
else
    fL = 1;
end
Fx0 = Fz*cx*lamda*fL/(1-lamda);
Fy0 = Fz*cy*tan(alpha)*fL/(1-lamda);
Fx = u*Fx0;
Fy = u*Fy0;

== matlab function Seven_dof2024a_DK/Tyer/pac2002/rr_dugoff ==
  data: Fz input; Fx0 output; u input; lamda input; alpha input; Fy0 output; Fx output; Fy output
function [Fx0,Fy0,Fx,Fy] = tire(Fz,u,lamda,alpha)
cx = -20;
cy = -20;
L = (1-lamda)/(2*sqrt((cx^2)*(lamda^2)+(cy^2)*((tan(alpha))^2)));
if L<1
    fL = L*(2-L);
else
    fL = 1;
end
Fx0 = Fz*cx*lamda*fL/(1-lamda);
Fy0 = Fz*cy*tan(alpha)*fL/(1-lamda);
Fx = u*Fx0;
Fy = u*Fy0;
